simulink model "Q4"  (R2021a)
settings: Solver=FixedStepAuto  StartTime=0.0  StopTime=20  FixedStep=0.001  RelTol=1e-3
values from neighbouring files (symbols this model uses):
  C = [cs1 0 0 -cs1 0 cs1*l1 0 ... (first row only)    [vibrtaion.m]
  K = [kt1+ks1 0 0 -ks1 0 ks1*l1 0 ... (first row only)    [vibrtaion.m]
  M = [m1 0   0  0  0  0  0 ... (first row only)    [vibrtaion.m]
settings Model: Creator=lenovo  LastModifiedBy=lenovo

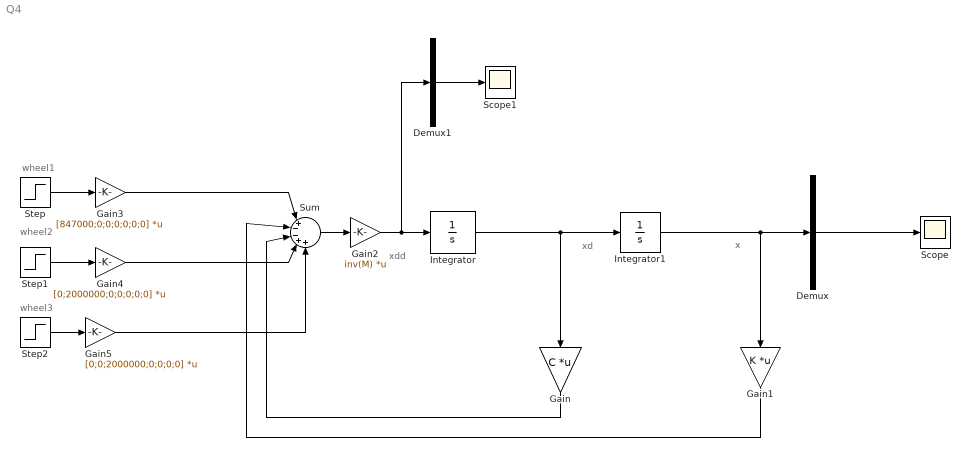
== system Q4 ==
  note: wheel3
  note: wheel2
  note: wheel1
  note: x
  note: xd
  note: xdd
  Demux : Demux  Outputs=7
  Demux1 : Demux  Outputs=7
  Gain : Gain  Gain=C  Multiplication=Matrix(K*u)
  Gain1 : Gain  Gain=K  Multiplication=Matrix(K*u)
  Gain2 : Gain  Gain=inv(M)  Multiplication=Matrix(K*u)
  Gain3 : Gain  Gain=[847000;0;0;0;0;0;0]  Multiplication=Matrix(K*u)
  Gain4 : Gain  Gain=[0;2000000;0;0;0;0;0]  Multiplication=Matrix(K*u)
  Gain5 : Gain  Gain=[0;0;2000000;0;0;0;0]  Multiplication=Matrix(K*u)
  Integrator : Integrator  InitialCondition=zeros(7,1)
  Integrator1 : Integrator  InitialCondition=zeros(7,1)
  Scope : Scope
  Scope1 : Scope
  Step : Step  Time=0  After=0.1  SampleTime=0
  Step1 : Step  Time=6/(20/3.6)  After=0.1  SampleTime=0
  Step2 : Step  Time=16.307/(20/3.6)  After=0.1  SampleTime=0
  Sum : Sum  Inputs=|+--++
  wires:
  Integrator/1 -> Gain/1, Integrator1/1
  Integrator1/1 -> Gain1/1, Demux/1
  Gain/1 -> Sum/3
  Gain1/1 -> Sum/2
  Sum/1 -> Gain2/1
  Gain2/1 -> Demux1/1, Integrator/1
  Step2/1 -> Gain5/1
  Step1/1 -> Gain4/1
  Step/1 -> Gain3/1
  Demux/4 -> Scope/1
  Gain3/1 -> Sum/1
  Gain4/1 -> Sum/4
  Gain5/1 -> Sum/5
  Demux1/4 -> Scope1/1
